simulink model "example_FanConst"  (R2018b)
settings: Solver=VariableStepAuto  StartTime=0.0  StopTime=240  RelTol=1e-3
undefined symbols (not defined in the file): density, Fan_Const
libraries: carnot x2
settings Model: Creator=drhf  LastModifiedBy=drhf

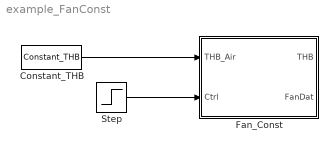
== system example_FanConst ==
  Constant_THB : carnot/Source/Simple/Constant_THB  t=20  mdot=0  p=1e5  mID=No Pressure Drop  fluid=Air  mix=0  mix2=0  mix3=0  dia=0.02  hgt=0
      settings: SourceProductName=Carnot
  Fan_Const : Subsystem  AncestorBlock=Fan_Const/Fan_Const  mask(Fan constant){Vdotmax=1000, dia=0.02, p0=101300, mix=0.01, Tini=20, UA=3, mcp=1000, e0=10, e1=10, e2=-1}
      mask prompts: Vdotmax "Vdotmax : volume flowrate in m³/h"; dia "diameter at in- and outlet [m]"; p0 "air pressure in Pa"; mix "kg of water per kg of dry air"; Tini "ambient and start temperature in °C"; UA "Thermal loss coefficient to ambient in W/K"; mcp "mcp: thermal capacity of the node in J/K"; e0 "e0: constant coefficient in W"; e1 "e1: linear coefficient in W*s/kg"; e2 "e2: quadratic coefficient in W*(s/kg)²"
      mask help:
      | Set constant volume flowrate according to the parameter Vdotmax and the control signal:
      | mdot = Vdotmax * Ctrl
      | Keep in mind that the flowrate in the THB is the massflowrate in kg/s whereas the parameters of the fan have different units.
      | Use the option "thermal node" if you want the pump to have thermal capacity and losses to ambient (or if you want to break an algebraic loop in the temperature signal).
      | Electric power is calculated Pel = e0 + e1*mdot + e2*mdot^2
      mask Help: web(fullfile(path_carnot('help'),'Pump_Const.html'),'-helpbrowser')
      mask TypeOptions dia: Pump_Const/dia
      mask TypeOptions mix: Pump_Const/mix
      mask TypeOptions Tini: Pump_Const/Tini
      mask TypeOptions UA: Pump_Const/UA
      mask TypeOptions mcp: Pump_Const/mcp
      mask TypeOptions e0: Pump_Const/e0
      mask TypeOptions e1: Pump_Const/e1
      mask TypeOptions e2: Pump_Const/e2
      mask DialogControl ParameterTabVar0 Prompt: Hydraulic
      mask DialogControl Container7 Prompt: Initial Values
      mask DialogControl ParameterTabVar012 Prompt: Thermal
      mask DialogControl ParameterTabVar01 Prompt: Electric
      mask Display:
      | plot(0,0,100,100,...
      |     [40,70,40,30,30,40,60,70,70,60,40],[70,50,30,40,60,70,70,60,40,30,30])
  Step : Step  Time=120  SampleTime=0
  wires:
  Constant_THB/1 -> Fan_Const/1(THB_Air)
  Step/1 -> Fan_Const/2(Ctrl)

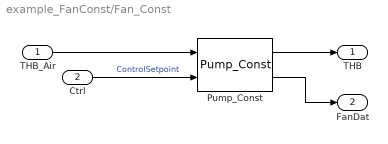
== system example_FanConst/Fan_Const ==
  THB_Air : Inport
  Ctrl : Inport  Port=2
  Pump_Const : carnot/Hydraulics/Pump_Const  mdotmax=Vdotmax/3600*density(Tini,p0,2,0)  dia=dia  p0=p0  fluid_id=Air  mix=mix  mix2=0  mix3=0  UA=UA  mcp=mcp  Tini=Tini  e0=e0  e1=e1  e2=e2
      settings: SourceProductName=Carnot
  THB : Outport
  FanDat : Outport  Port=2
  wires:
  THB_Air/1 -> Pump_Const/1
  Ctrl/1 -> Pump_Const/2  "ControlSetpoint"
  Pump_Const/1 -> THB/1
  Pump_Const/2 -> FanDat/1
